simulink model "constants2019bwithfunction2019b2019b"  (R2020a)
settings: Solver=VariableStepAuto  StartTime=0.0  StopTime=inf  RelTol=1e-3
undefined symbols (not defined in the file): f
libraries: instrumentlib x15, dspnetwork x12
settings Model: Creator=Jskyl  LastModifiedBy=Jskyl
settings DebuggingCC: ArithmeticOperatorsInVariantConditions=warning
settings SFSimCC: CustomCodeUndefinedFunction=UseInterfaceOnly

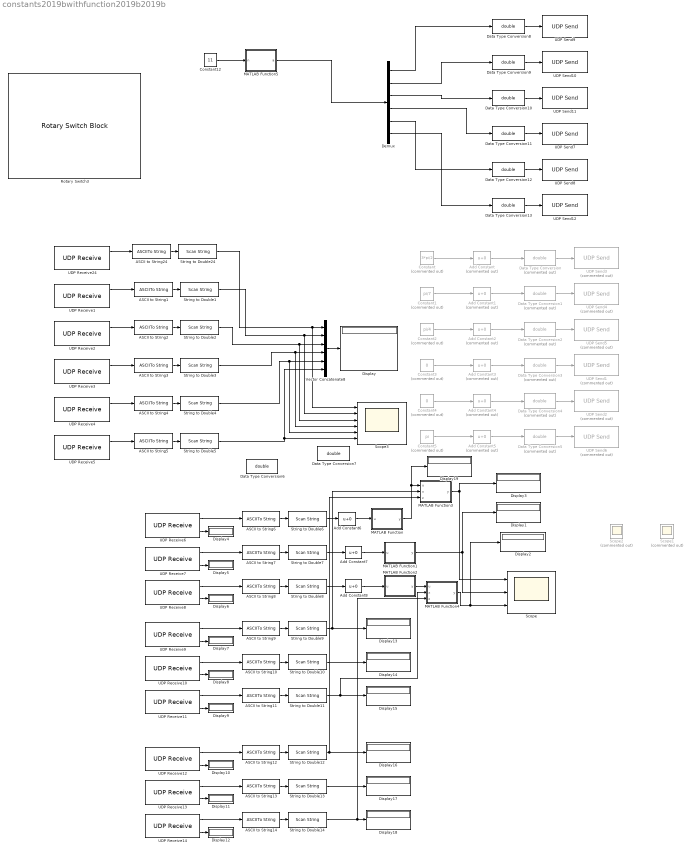
== system constants2019bwithfunction2019b2019b ==
  ASCII to String{1..14,24} (15 alike) : ASCIIToString
  Add Constant{,1..5} (6 alike) : Bias  Commented=on
  Add Constant6 : Bias
  Add Constant7 : Bias
  Add Constant8 : Bias
  Constant : Constant  Commented=on  Value=3*pi/2
  Constant1 : Constant  Commented=on  Value=pi/7
  Constant12 : Constant  Value=11
  Constant2 : Constant  Commented=on  Value=pi/4
  Constant3 : Constant  Commented=on  Value=0
  Constant4 : Constant  Commented=on  Value=0
  Constant5 : Constant  Commented=on  Value=pi
  Data Type Conversion{,1..5} (6 alike) : DataTypeConversion  Commented=on  OutDataTypeStr=double  ConvertRealWorld=Stored Integer (SI)
  Data Type Conversion{7..13} (7 alike) : DataTypeConversion  OutDataTypeStr=double  ConvertRealWorld=Stored Integer (SI)
  Data Type Conversion6 : DataTypeConversion  OutDataTypeStr=double  RndMeth=Round
  Demux : Demux  Outputs=6
  Display{,1..19} (20 alike) : Display
      Display10 settings: Format=bank
      Display11 settings: Format=bank
      Display12 settings: Format=bank
      Display4 settings: Format=bank
      Display5 settings: Format=bank
      Display6 settings: Format=bank
      Display7 settings: Format=bank
      Display8 settings: Format=bank
      Display9 settings: Format=bank
  MATLAB Function : MATLAB Function  TreatAsAtomicUnit=on
  MATLAB Function1 : MATLAB Function  TreatAsAtomicUnit=on
  MATLAB Function2 : MATLAB Function  TreatAsAtomicUnit=on
  MATLAB Function3 : MATLAB Function  TreatAsAtomicUnit=on
  MATLAB Function4 : MATLAB Function  TreatAsAtomicUnit=on
  MATLAB Function5 : MATLAB Function  TreatAsAtomicUnit=on
  Rotary Switch3 : RotarySwitchBlock
      settings: Values={{'Up', 'Down', 'In', 'out', 'Left', 'Right', 'Rest'}, [11 21 31 41 51 61 72]}
  Scope : Scope  NumInputPorts=3
  Scope1 : Scope  Commented=on
  Scope2 : Scope  Commented=on
  Scope3 : Scope  NumInputPorts=6
  String to Double{1..14,24} (15 alike) : ScanString  Format="\"%lf\""
  UDP Receive1 : instrumentlib/UDP Receive  Host=localhost  Port=2002  LocalPort=2002  EnablePortSharing=off  GetLatestData=on  DataSize="[1  5]"  DataType=uint8  ASCIIFormatting=%f,  Terminator=LF  ByteOrder=BigEndian  EnableBlockingMode=off  Timeout=10  SampleTime=0.01  LocalAddress=127.0.0.1
  UDP Receive10 : instrumentlib/UDP Receive  Host=localhost  Port=6200  LocalPort=6200  EnablePortSharing=off  GetLatestData=on  DataSize="[1  1]"  DataType=uint8  ASCIIFormatting=%f,  Terminator=LF  ByteOrder=BigEndian  EnableBlockingMode=off  Timeout=10  SampleTime=0.02  LocalAddress=127.0.0.1
  UDP Receive11 : instrumentlib/UDP Receive  Host=localhost  Port=6300  LocalPort=6300  EnablePortSharing=off  GetLatestData=on  DataSize="[1  1]"  DataType=uint8  ASCIIFormatting=%f,  Terminator=LF  ByteOrder=BigEndian  EnableBlockingMode=off  Timeout=10  SampleTime=0.02  LocalAddress=127.0.0.1
  UDP Receive12 : instrumentlib/UDP Receive  Host=localhost  Port=7100  LocalPort=7100  EnablePortSharing=off  GetLatestData=on  DataSize="[1  1]"  DataType=uint8  ASCIIFormatting=%f,  Terminator=LF  ByteOrder=BigEndian  EnableBlockingMode=off  Timeout=10  SampleTime=0.02  LocalAddress=127.0.0.1
  UDP Receive13 : instrumentlib/UDP Receive  Host=localhost  Port=7200  LocalPort=7200  EnablePortSharing=off  GetLatestData=on  DataSize="[1  1]"  DataType=uint8  ASCIIFormatting=%f,  Terminator=LF  ByteOrder=BigEndian  EnableBlockingMode=off  Timeout=10  SampleTime=0.02  LocalAddress=127.0.0.1
  UDP Receive14 : instrumentlib/UDP Receive  Host=localhost  Port=7300  LocalPort=7300  EnablePortSharing=off  GetLatestData=on  DataSize="[1  1]"  DataType=uint8  ASCIIFormatting=%f,  Terminator=LF  ByteOrder=BigEndian  EnableBlockingMode=off  Timeout=10  SampleTime=0.02  LocalAddress=127.0.0.1
  UDP Receive2 : instrumentlib/UDP Receive  Host=localhost  Port=2003  LocalPort=2003  EnablePortSharing=off  GetLatestData=on  DataSize="[1  5]"  DataType=uint8  ASCIIFormatting=%f,  Terminator=LF  ByteOrder=BigEndian  EnableBlockingMode=off  Timeout=10  SampleTime=0.01  LocalAddress=127.0.0.1
  UDP Receive24 : instrumentlib/UDP Receive  Host=localhost  Port=2001  LocalPort=2001  EnablePortSharing=off  GetLatestData=on  DataSize="[1  5]"  DataType=uint8  ASCIIFormatting=%f,  Terminator=LF  ByteOrder=BigEndian  EnableBlockingMode=off  Timeout=10  SampleTime=0.01  LocalAddress=127.0.0.1
  UDP Receive3 : instrumentlib/UDP Receive  Host=localhost  Port=2004  LocalPort=2004  EnablePortSharing=off  GetLatestData=on  DataSize="[1  5]"  DataType=uint8  ASCIIFormatting=%f,  Terminator=LF  ByteOrder=BigEndian  EnableBlockingMode=off  Timeout=10  SampleTime=0.01  LocalAddress=127.0.0.1
  UDP Receive4 : instrumentlib/UDP Receive  Host=localhost  Port=2005  LocalPort=2005  EnablePortSharing=off  GetLatestData=on  DataSize="[1  5]"  DataType=uint8  ASCIIFormatting=%f,  Terminator=LF  ByteOrder=BigEndian  EnableBlockingMode=off  Timeout=10  SampleTime=0.01  LocalAddress=127.0.0.1
  UDP Receive5 : instrumentlib/UDP Receive  Host=localhost  Port=2006  LocalPort=2006  EnablePortSharing=off  GetLatestData=on  DataSize="[1  5]"  DataType=uint8  ASCIIFormatting=%f,  Terminator=LF  ByteOrder=BigEndian  EnableBlockingMode=off  Timeout=10  SampleTime=0.01  LocalAddress=127.0.0.1
  UDP Receive6 : instrumentlib/UDP Receive  Host=localhost  Port=5100  LocalPort=5100  EnablePortSharing=off  GetLatestData=on  DataSize="[1  7]"  DataType=uint8  ASCIIFormatting=%f,  Terminator=LF  ByteOrder=BigEndian  EnableBlockingMode=off  Timeout=10  SampleTime=0.02  LocalAddress=127.0.0.1
  UDP Receive7 : instrumentlib/UDP Receive  Host=localhost  Port=5200  LocalPort=5200  EnablePortSharing=off  GetLatestData=on  DataSize="[1  6]"  DataType=uint8  ASCIIFormatting=%f,  Terminator=LF  ByteOrder=BigEndian  EnableBlockingMode=off  Timeout=10  SampleTime=0.02  LocalAddress=127.0.0.1
  UDP Receive8 : instrumentlib/UDP Receive  Host=localhost  Port=5300  LocalPort=5300  EnablePortSharing=off  GetLatestData=on  DataSize="[1  7]"  DataType=uint8  ASCIIFormatting=%f,  Terminator=LF  ByteOrder=BigEndian  EnableBlockingMode=off  Timeout=10  SampleTime=0.02  LocalAddress=127.0.0.1
  UDP Receive9 : instrumentlib/UDP Receive  Host=localhost  Port=6100  LocalPort=6100  EnablePortSharing=off  GetLatestData=on  DataSize="[1  1]"  DataType=uint8  ASCIIFormatting=%f,  Terminator=LF  ByteOrder=BigEndian  EnableBlockingMode=off  Timeout=10  SampleTime=0.02  LocalAddress=127.0.0.1
  UDP Send1 : dspnetwork/UDP Send  Commented=on  remoteURL='127.0.0.1'  remotePort=3004  localURL='0.0.0.0'  localPortSource=Automatically determine  localPort=-1  sendBufferSize=8192  sampletime=-1  blockPlatform=[]  separateLengthPort=0
  UDP Send10 : dspnetwork/UDP Send  remoteURL='127.0.0.1'  remotePort=3002  localURL='0.0.0.0'  localPortSource=Automatically determine  localPort=-1  sendBufferSize=8192  sampletime=-1  blockPlatform=[]  separateLengthPort=0
  UDP Send11 : dspnetwork/UDP Send  remoteURL='127.0.0.1'  remotePort=3003  localURL='0.0.0.0'  localPortSource=Automatically determine  localPort=-1  sendBufferSize=8192  sampletime=-1  blockPlatform=[]  separateLengthPort=0
  UDP Send12 : dspnetwork/UDP Send  remoteURL='127.0.0.1'  remotePort=3006  localURL='0.0.0.0'  localPortSource=Automatically determine  localPort=-1  sendBufferSize=8192  sampletime=-1  blockPlatform=[]  separateLengthPort=0
  UDP Send2 : dspnetwork/UDP Send  Commented=on  remoteURL='127.0.0.1'  remotePort=3005  localURL='0.0.0.0'  localPortSource=Automatically determine  localPort=-1  sendBufferSize=8192  sampletime=-1  blockPlatform=[]  separateLengthPort=0
  UDP Send3 : dspnetwork/UDP Send  Commented=on  remoteURL='127.0.0.1'  remotePort=3001  localURL='0.0.0.0'  localPortSource=Automatically determine  localPort=-1  sendBufferSize=8192  sampletime=-1  blockPlatform=[]  separateLengthPort=0
  UDP Send4 : dspnetwork/UDP Send  Commented=on  remoteURL='127.0.0.1'  remotePort=3002  localURL='0.0.0.0'  localPortSource=Automatically determine  localPort=-1  sendBufferSize=8192  sampletime=-1  blockPlatform=[]  separateLengthPort=0
  UDP Send5 : dspnetwork/UDP Send  Commented=on  remoteURL='127.0.0.1'  remotePort=3003  localURL='0.0.0.0'  localPortSource=Automatically determine  localPort=-1  sendBufferSize=8192  sampletime=-1  blockPlatform=[]  separateLengthPort=0
  UDP Send6 : dspnetwork/UDP Send  Commented=on  remoteURL='127.0.0.1'  remotePort=3006  localURL='0.0.0.0'  localPortSource=Automatically determine  localPort=-1  sendBufferSize=8192  sampletime=-1  blockPlatform=[]  separateLengthPort=0
  UDP Send7 : dspnetwork/UDP Send  remoteURL='127.0.0.1'  remotePort=3004  localURL='0.0.0.0'  localPortSource=Automatically determine  localPort=-1  sendBufferSize=8192  sampletime=-1  blockPlatform=[]  separateLengthPort=0
  UDP Send8 : dspnetwork/UDP Send  remoteURL='127.0.0.1'  remotePort=3005  localURL='0.0.0.0'  localPortSource=Automatically determine  localPort=-1  sendBufferSize=8192  sampletime=-1  blockPlatform=[]  separateLengthPort=0
  UDP Send9 : dspnetwork/UDP Send  remoteURL='127.0.0.1'  remotePort=3001  localURL='0.0.0.0'  localPortSource=Automatically determine  localPort=-1  sendBufferSize=8192  sampletime=-1  blockPlatform=[]  separateLengthPort=0
  Vector Concatenate8 : Concatenate  NumInputs=6
  wires:
  Data Type Conversion/1 -> UDP Send3/1
  Data Type Conversion5/1 -> UDP Send6/1
  Data Type Conversion4/1 -> UDP Send2/1
  Data Type Conversion1/1 -> UDP Send4/1
  Data Type Conversion3/1 -> UDP Send1/1
  Data Type Conversion2/1 -> UDP Send5/1
  Constant/1 -> Add Constant/1
  Constant1/1 -> Add Constant1/1
  Constant2/1 -> Add Constant2/1
  Constant3/1 -> Add Constant3/1
  Constant4/1 -> Add Constant4/1
  Constant5/1 -> Add Constant5/1
  Add Constant3/1 -> Data Type Conversion3/1
  Add Constant/1 -> Data Type Conversion/1
  Add Constant1/1 -> Data Type Conversion1/1
  Add Constant2/1 -> Data Type Conversion2/1
  Add Constant5/1 -> Data Type Conversion5/1
  Add Constant4/1 -> Data Type Conversion4/1
  ASCII to String24/1 -> String to Double24/1
  ASCII to String1/1 -> String to Double1/1
  UDP Receive1/1 -> ASCII to String1/1
  ASCII to String2/1 -> String to Double2/1
  UDP Receive2/1 -> ASCII to String2/1
  ASCII to String3/1 -> String to Double3/1
  UDP Receive3/1 -> ASCII to String3/1
  ASCII to String4/1 -> String to Double4/1
  UDP Receive4/1 -> ASCII to String4/1
  ASCII to String5/1 -> String to Double5/1
  UDP Receive5/1 -> ASCII to String5/1
  Vector Concatenate8/1 -> Display/1
  String to Double1/1 -> Scope3/2, Vector Concatenate8/2
  String to Double2/1 -> Scope3/3, Vector Concatenate8/3
  String to Double3/1 -> Scope3/4, Vector Concatenate8/4
  String to Double4/1 -> Scope3/5, Vector Concatenate8/5
  String to Double5/1 -> Vector Concatenate8/6, Scope3/6
  UDP Receive24/1 -> ASCII to String24/1
  String to Double24/1 -> Scope3/1, Vector Concatenate8/1
  ASCII to String7/1 -> String to Double7/1
  UDP Receive7/1 -> ASCII to String7/1
  ASCII to String8/1 -> String to Double8/1
  UDP Receive8/1 -> ASCII to String8/1
  String to Double8/1 -> Add Constant8/1
  String to Double7/1 -> Add Constant7/1
  ASCII to String6/1 -> String to Double6/1
  String to Double6/1 -> Add Constant6/1
  UDP Receive6/1 -> ASCII to String6/1
  UDP Receive6/2 -> Display4/1
  UDP Receive7/2 -> Display5/1
  UDP Receive8/2 -> Display6/1
  Add Constant8/1 -> MATLAB Function2/1(u)
  Add Constant7/1 -> MATLAB Function1/1(u)
  MATLAB Function1/1(y) -> Scope/2, Display1/1
  UDP Receive10/2 -> Display8/1
  UDP Receive9/1 -> ASCII to String9/1
  ASCII to String11/1 -> String to Double11/1
  ASCII to String10/1 -> String to Double10/1
  ASCII to String9/1 -> String to Double9/1
  UDP Receive11/2 -> Display9/1
  UDP Receive10/1 -> ASCII to String10/1
  UDP Receive9/2 -> Display7/1
  UDP Receive11/1 -> ASCII to String11/1
  UDP Receive13/2 -> Display11/1
  UDP Receive12/1 -> ASCII to String12/1
  ASCII to String14/1 -> String to Double14/1
  ASCII to String13/1 -> String to Double13/1
  ASCII to String12/1 -> String to Double12/1
  UDP Receive14/2 -> Display12/1
  UDP Receive13/1 -> ASCII to String13/1
  UDP Receive12/2 -> Display10/1
  UDP Receive14/1 -> ASCII to String14/1
  String to Double10/1 -> Display14/1
  String to Double11/1 -> MATLAB Function4/2(x), Display15/1
  String to Double13/1 -> Display17/1
  String to Double14/1 -> MATLAB Function4/3(z), Display18/1
  String to Double9/1 -> Display13/1, MATLAB Function3/2(x)
  Add Constant6/1 -> MATLAB Function/1(u)
  MATLAB Function3/1(y) -> Display3/1, Scope/1
  String to Double12/1 -> Display16/1, MATLAB Function3/3(z)
  MATLAB Function/1(y) -> Display19/1, MATLAB Function3/1(u)
  MATLAB Function2/1(y) -> MATLAB Function4/1(u)
  MATLAB Function4/1(y) -> Display2/1, Scope/3
  Data Type Conversion13/1 -> UDP Send12/1
  Data Type Conversion9/1 -> UDP Send10/1
  Data Type Conversion12/1 -> UDP Send8/1
  Data Type Conversion11/1 -> UDP Send7/1
  Data Type Conversion10/1 -> UDP Send11/1
  Data Type Conversion8/1 -> UDP Send9/1
  Constant12/1 -> MATLAB Function5/1(n)
  Demux/6 -> Data Type Conversion13/1
  Demux/5 -> Data Type Conversion12/1
  Demux/4 -> Data Type Conversion11/1
  Demux/3 -> Data Type Conversion10/1
  Demux/2 -> Data Type Conversion9/1
  Demux/1 -> Data Type Conversion8/1
  MATLAB Function5/1(a) -> Demux/1

== matlab function constants2019bwithfunction2019b2019b/MATLAB Function ==
  data: u input; y output
function y = fcn(u)

if u > 1
    c = sprintf('%f', u);
    y = str2double(c(2:6));
    %disp(y);
else
    y = u;
end

== matlab function constants2019bwithfunction2019b2019b/MATLAB Function2 ==
  data: u input; y output
function y = fcn(u)

if u > 1
    c = sprintf('%f', u);
    y = str2double(c(2:6));
    disp(y);
else
    y = u;
end

== matlab function constants2019bwithfunction2019b2019b/MATLAB Function3 ==
  data: u input; y output; x input; z input
function y = fcn(u, x, z)

if z == 1
    if u < 1
        %c = sprintf('%f', u);
        y = x + u;
        disp(y);
    else
        y = u;
    end
else
    y = u;
end

== matlab function constants2019bwithfunction2019b2019b/MATLAB Function4 ==
  data: u input; y output; x input; z input
function y = fcn(u, x, z)

if z == 1
    if u < 1
        %c = sprintf('%f', u);
        y = x + u;
        disp(y);
    else
        y = u;
    end
else
    y = u;
end

== matlab function constants2019bwithfunction2019b2019b/MATLAB Function5 ==
  data: n input; a output
function a = Pos(n)
% n = input('Enter a number: ');
  
switch n
  
    case 11
        a=[pi, pi,  pi, 0, 0, pi]; % up
    case 21
        a=[3*pi/2, pi/7, pi/4, 0, 0, pi]; % down
    case 31
        a=[pi/2, 3*pi/2, pi, 0, 0, pi]; % in
    case 41
        a=[pi/2, pi/2, pi, 0, 0,  pi]; % out
    case 51
        a=[pi, 3*pi/2, pi, 0, 0, pi]; % left
    case 61
        a=[pi, pi/2, pi, 0, 0, pi]; % right
    case 71
        a=[0.2,-0.1,-0.3, 0, 0, pi]; % rest
    otherwise
        a=[0.2,-0.1,-0.3, 0, 0, pi]; % rest
end

%{
case 11
        a=[0.2,-0.1,-0.3]; % up
    case 21
        a=[-0.01,-0.1,-0.3]; % down
    case 31
        a=[0.2,0.27,-0.3]; % in
    case 41
        a=[0,0,0.1]; % out
    case 51
        a=[-0.2,0.1,-0.2]; % left
    case 61
        a=[0.2,-0.1,0.2]; % right
    case 71
        a=[0.2,-0.1,-0.3]; % rest
    otherwise
        a=[0.2,-0.1,-0.3]; % rest
end
%}

== matlab function constants2019bwithfunction2019b2019b/MATLAB Function1 ==
  data: u input; y output
function y = fcn(u)

if u > 10
    c = sprintf('%f', u);
    y = str2double(c(2:6));
    disp(y);
else
    y = u;
end
